simulink model "Joystick"  (R2023a)
settings: Solver=FixedStepDiscrete  StartTime=0.0  StopTime=inf  RelTol=1e-3
values from neighbouring files (symbols this model uses):
  stopSimulationFlag = 0    [InitializeModelForTest.m]
undefined symbols (not defined in the file or in its folder): ComPortTransmitData, NULL, pitchBoundary, rollBoundary, throttleBoundary, yawBoundary
libraries: instrumentseriallib x6, aerolibanimutils x5
settings Model: Creator=admin  LastModifiedBy=ASUS
settings OptimizationCC: DefaultParameterBehavior=Inlined  UseDivisionForNetSlopeComputation=on  GainParamInheritBuiltInType=on  UseFloatMulNetSlope=on  InlineInvariantSignals=on  PassReuseOutputArgsAs=Individual arguments  ZeroExternalMemoryAtStartup=off  ZeroInternalMemoryAtStartup=off  NoFixptDivByZeroProtection=on  EfficientFloat2IntCast=on  LifeSpan=1  OptimizeBlockOrder=speed  DifferentSizesBufferReuse=on  EfficientTunableParamExpr=on
settings DebuggingCC: ParameterTunabilityLossMsg=error  SFUnexpectedBacktrackingDiag=warning  SFNoUnconditionalDefaultTransitionDiag=warning
settings HardwareCC: ProdBitPerPointer=32  ProdBitPerSizeT=32  ProdBitPerPtrDiffT=32  ProdLargestAtomicInteger=Long  ProdLargestAtomicFloat=Double  ProdWordSize=32  ProdLongLongMode=on  ProdHWDeviceType=ARM Compatible->ARM Cortex-M  TargetBitPerPointer=64  TargetBitPerSizeT=64  TargetBitPerPtrDiffT=64  TargetLongLongMode=on  TargetIntDivRoundTo=Zero  TargetEndianess=LittleEndian  TargetWordSize=64  TargetHWDeviceType=MATLAB Host  ProdEqTarget=off
settings SFSimCC: MATLABDynamicMemAlloc=off
settings RTWCC: Description=Embedded Coder  SystemTargetFile=ert.tlc  TemplateMakefile=ert_default_tmf  GenerateReport=on  BuildConfiguration=Debug  LaunchReport=on
settings CodeAppCC: ForceParamTrailComments=on  IgnoreCustomStorageClasses=off  OperatorAnnotations=on  SimulinkDataObjDesc=on  SFDataObjDesc=on  CustomSymbolStrGlobalVar=rt$N$M  CustomSymbolStrType=$N$M  CustomSymbolStrFcn=$N$M$F  CustomSymbolStrMacro=$N$M  InsertBlockDesc=on  EnableCustomComments=on
settings ERTTargetCC: TargetLangStandard=C99 (ISO)  GenerateSampleERTMain=on  IncludeMdlTerminateFcn=off  CombineSignalStateStructs=on  SupportAbsoluteTime=off  SupportComplex=off  SupportNonInlinedSFcns=on  InlinedParameterPlacement=NonHierarchical  ERTCustomFileTemplate=example_file_process.tlc  ERTFilePackagingFormat=CompactWithDataFile

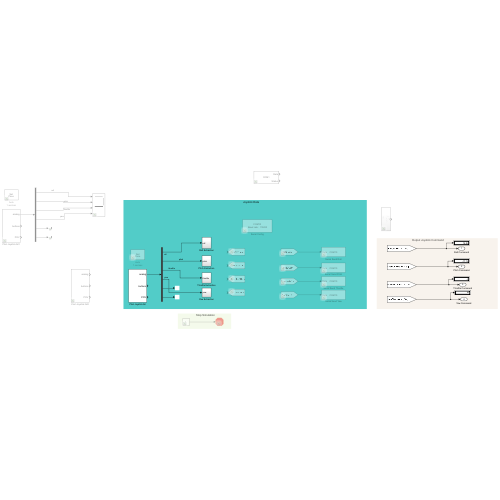
[thumbnail: Simulink's stored preview of the top-level diagram]
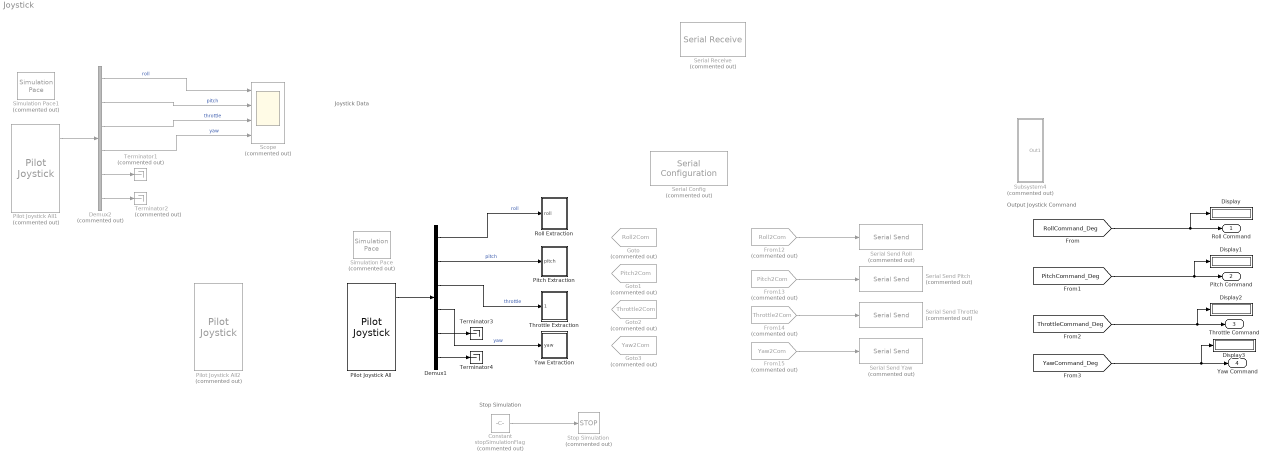
== system Joystick ==
  note: Joystick Data
  note: Output Joystick Command
  note: Stop Simulation
  Constant : Constant  Commented=on  Value=stopSimulationFlag
  Demux1 : Demux  Outputs=6
  Demux2 : Demux  Commented=on  Outputs=6
  Display{,1..3} (4 alike) : Display
  From12 : From  Commented=on  GotoTag=Roll2Com  TagVisibility=global
  From13 : From  Commented=on  GotoTag=Pitch2Com  TagVisibility=global
  From14 : From  Commented=on  GotoTag=Throttle2Com  TagVisibility=global
  From15 : From  Commented=on  GotoTag=Yaw2Com  TagVisibility=global
  Goto : Goto  Commented=on  GotoTag=Roll2Com  TagVisibility=global
  Goto1 : Goto  Commented=on  GotoTag=Pitch2Com  TagVisibility=global
  Goto2 : Goto  Commented=on  GotoTag=Throttle2Com  TagVisibility=global
  Goto3 : Goto  Commented=on  GotoTag=Yaw2Com  TagVisibility=global
  Pilot Joystick All : aerolibanimutils/Pilot Joystick  JoystickID=Joystick1  OutputConfiguration=AllOutputs  SampleTime=1/50
      settings: LibrarySourceBlock=aerolibanimutils/Pilot Joystick All
  Pilot Joystick All1 : aerolibanimutils/Pilot Joystick  Commented=on  JoystickID=Joystick1  OutputConfiguration=AllOutputs  SampleTime=1/50
      settings: LibrarySourceBlock=aerolibanimutils/Pilot Joystick All
  Pilot Joystick All2 : aerolibanimutils/Pilot Joystick  Commented=on  JoystickID=Joystick1  OutputConfiguration=AllOutputs  SampleTime=1/50
      settings: LibrarySourceBlock=aerolibanimutils/Pilot Joystick All
  Pitch Extraction : Subsystem
  Roll Extraction : Subsystem
  Scope : Scope  Commented=on  NumInputPorts=4
  Serial Config : instrumentseriallib/Serial Configuration  Priority=-200000  Commented=on  PortSel=COM10  Port=COM10  ComPort=COM10  BaudRate=115200  DataBits=8  Parity=none  StopBits=1  ByteOrder=little-endian  FlowControl=none  Timeout=10  SimulateUsing=Interpreted execution  BlockInModel=on  aMode=1
  Serial Receive : instrumentseriallib/Serial Receive  Priority=1  Commented=on  PortSel=COM1  Port=COM1  ComPort=COM1  DataType=uint8  SaveDataType=uint8  ToggleHeader=on  Header=[]  ToggleTerminator=on  Terminator=<none>  CustomTerminator=[]  InputFormat=Column major  ToggleDataSize=on  DataSize=[1 1]  EnableBlockingMode=off  ActionDataUnavailable=Output last received value  ActionWhenDataUnavailable=Output last received value  CustomValue=0  SampleTime=0.01  SimulateUsing=Interpreted execution  BlockInModel=on  aMode=1
      settings: LibrarySourceBlock=embeddedtargetslib/Host Communication/Serial Receive
  Serial Send Pitch : instrumentseriallib/Serial Send  Priority=1  Commented=on  PortSel=COM10  Port=COM10  ComPort=COM10  Header=['P']  Terminator=NULL ('\0')  CustomTerminator=[' ']  EnableBlockingMode=off  SimulateUsing=Interpreted execution  BlockInModel=on  aMode=1
  Serial Send Roll : instrumentseriallib/Serial Send  Priority=1  Commented=on  PortSel=COM10  Port=COM10  ComPort=COM10  Header=['R']  Terminator=NULL ('\0')  CustomTerminator=[' ']  EnableBlockingMode=off  SimulateUsing=Interpreted execution  BlockInModel=on  aMode=1
  Serial Send Throttle : instrumentseriallib/Serial Send  Priority=1  Commented=on  PortSel=COM10  Port=COM10  ComPort=COM10  Header=['T']  Terminator=NULL ('\0')  CustomTerminator=[' ']  EnableBlockingMode=off  SimulateUsing=Interpreted execution  BlockInModel=on  aMode=1
  Serial Send Yaw : instrumentseriallib/Serial Send  Priority=1  Commented=on  PortSel=COM10  Port=COM10  ComPort=COM10  Header=['Y']  Terminator=NULL ('\0')  CustomTerminator=[' ']  EnableBlockingMode=off  SimulateUsing=Interpreted execution  BlockInModel=on  aMode=1
  Simulation Pace : aerolibanimutils/Simulation Pace  Commented=on  SimulationPace=1  SleepMode=Auto  OutputPaceError=off  SampleTime=1/50
  Simulation Pace1 : aerolibanimutils/Simulation Pace  Commented=on  SimulationPace=1  SleepMode=Auto  OutputPaceError=off  SampleTime=1/50
  Stop Simulation : Stop  Commented=on
  Subsystem4 : Subsystem  Commented=on
  Terminator1 : Terminator  Commented=on
  Terminator2 : Terminator  Commented=on
  Terminator3 : Terminator
  Terminator4 : Terminator
  Throttle Extraction : Subsystem
  Yaw Extraction : Subsystem
  Roll Command : Outport
  Pitch Command : Outport  Port=2
  Throttle Command : Outport  Port=3
  Yaw Command : Outport  Port=4
  wires:
  Demux1/6 -> Terminator4/1
  Demux1/5 -> Terminator3/1
  Pilot Joystick All/1 -> Demux1/1
  Demux1/2 -> Pitch Extraction/1(pitch)  "pitch"
  Demux1/3 -> Throttle Extraction/1(throttle)  "throttle"
  Demux1/4 -> Yaw Extraction/1(yaw)  "yaw"
  Constant/1 -> Stop Simulation/1
  [PitchCommand_Deg] -> Display1/1, Pitch Command/1
  [ThrottleCommand_Deg] -> Display2/1, Throttle Command/1
  [YawCommand_Deg] -> Display3/1, Yaw Command/1
  [RollCommand_Deg] -> Display/1, Roll Command/1
  From12/1 -> Serial Send Roll/1
  From13/1 -> Serial Send Pitch/1
  From14/1 -> Serial Send Throttle/1
  From15/1 -> Serial Send Yaw/1
  Demux2/4 -> Scope/4  "yaw"
  Demux2/3 -> Scope/3  "throttle"
  Demux2/2 -> Scope/2  "pitch"
  Demux2/1 -> Scope/1  "roll"
  Pilot Joystick All1/1 -> Demux2/1
  Demux2/5 -> Terminator1/1
  Demux2/6 -> Terminator2/1
  Demux1/1 -> Roll Extraction/1(roll)  "roll"

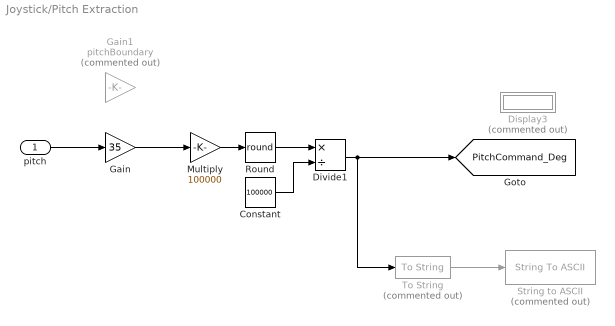
== system Joystick/Pitch Extraction ==
  pitch : Inport
  Constant : Constant  Value=100000
  Display3 : Display  Commented=on
  Divide1 : Product  Inputs=*/
  Gain : Gain  Gain=35
  Gain1 : Gain  Commented=on  Gain=pitchBoundary
  Multiply : Gain  Gain=100000
  Round : Rounding  Operator=round
  String to ASCII : StringToASCII  Commented=on  OutputVectorSize=8
  To String : ToString  Commented=on
  tag scope: PitchCommand_Deg=global
  wires:
  pitch/1 -> Gain/1
  To String/1 -> String to ASCII/1
  Multiply/1 -> Round/1
  Constant/1 -> Divide1/2
  Round/1 -> Divide1/1
  Gain/1 -> Multiply/1
  Divide1/1 -> [PitchCommand_Deg], To String/1

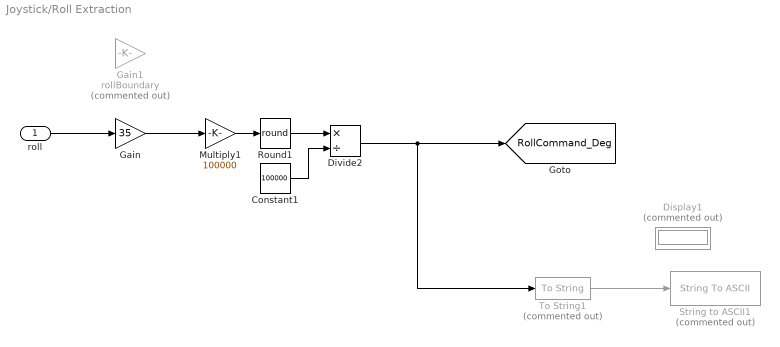
== system Joystick/Roll Extraction ==
  roll : Inport
  Constant1 : Constant  Value=100000
  Display1 : Display  Commented=on
  Divide2 : Product  Inputs=*/
  Gain : Gain  Gain=35
  Gain1 : Gain  Commented=on  Gain=rollBoundary
  Multiply1 : Gain  Gain=100000
  Round1 : Rounding  Operator=round
  String to ASCII1 : StringToASCII  Commented=on  OutputVectorSize=8
  To String1 : ToString  Commented=on
  tag scope: RollCommand_Deg=global
  wires:
  roll/1 -> Gain/1
  Divide2/1 -> [RollCommand_Deg], To String1/1
  Round1/1 -> Divide2/1
  Multiply1/1 -> Round1/1
  Constant1/1 -> Divide2/2
  To String1/1 -> String to ASCII1/1
  Gain/1 -> Multiply1/1

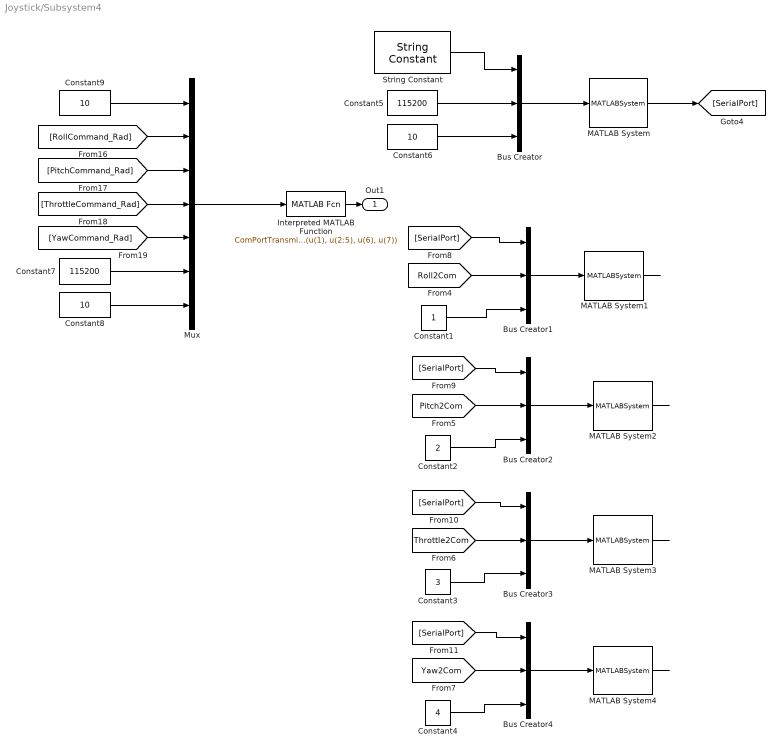
== system Joystick/Subsystem4 ==
  Bus Creator{,1..4} (5 alike) : BusCreator  Inputs=3
  Constant1 : Constant
  Constant2 : Constant  Value=2
  Constant3 : Constant  Value=3
  Constant4 : Constant  Value=4
  Constant5 : Constant  Value=115200
  Constant6 : Constant  Value=10
  Constant7 : Constant  Value=115200
  Constant8 : Constant  Value=10
  Constant9 : Constant  Value=10
  Interpreted MATLAB Function : MATLABFcn  MATLABFcn=ComPortTransmitData(u(1), u(2:5), u(6), u(7))
  MATLAB System : MATLABSystem  System=PortConfig  SimulateUsing=Code generation
      mask Type: PortConfig
      mask Display:
      | disp('PortConfig');
      | port_label('input',1,'u');
      | port_label('output',1,'y');
  MATLAB System{1..4} (4 alike) : MATLABSystem  System=SerialSend  SimulateUsing=Code generation
      mask Type: SerialSend
      mask Display:
      | disp('SerialSend');
      | port_label('input',1,'u');
      | port_label('output',1,'y');
  Mux : Mux  Inputs=7
  String Constant : StringConstant  String="\"COM10\""
  Out1 : Outport
  wires:
  [Yaw2Com] -> Bus Creator4/2
  Constant5/1 -> Bus Creator/2
  [PitchCommand_Rad] -> Mux/3
  MATLAB System4/1 -> ?
  [SerialPort] -> Bus Creator3/1
  Interpreted MATLAB Function/1 -> Out1/1
  Bus Creator2/1 -> MATLAB System2/1
  [Roll2Com] -> Bus Creator1/2
  Constant4/1 -> Bus Creator4/3
  Bus Creator/1 -> MATLAB System/1
  [SerialPort] -> Bus Creator4/1
  Bus Creator1/1 -> MATLAB System1/1
  [SerialPort] -> Bus Creator2/1
  MATLAB System1/1 -> ?
  MATLAB System3/1 -> ?
  [Throttle2Com] -> Bus Creator3/2
  Constant8/1 -> Mux/7
  MATLAB System/1 -> [SerialPort]
  String Constant/1 -> Bus Creator/1
  [RollCommand_Rad] -> Mux/2
  Bus Creator4/1 -> MATLAB System4/1
  Mux/1 -> Interpreted MATLAB Function/1
  Constant9/1 -> Mux/1
  Constant6/1 -> Bus Creator/3
  Bus Creator3/1 -> MATLAB System3/1
  MATLAB System2/1 -> ?
  Constant2/1 -> Bus Creator2/3
  Constant1/1 -> Bus Creator1/3
  Constant7/1 -> Mux/6
  [Pitch2Com] -> Bus Creator2/2
  [YawCommand_Rad] -> Mux/5
  [ThrottleCommand_Rad] -> Mux/4
  Constant3/1 -> Bus Creator3/3
  [SerialPort] -> Bus Creator1/1

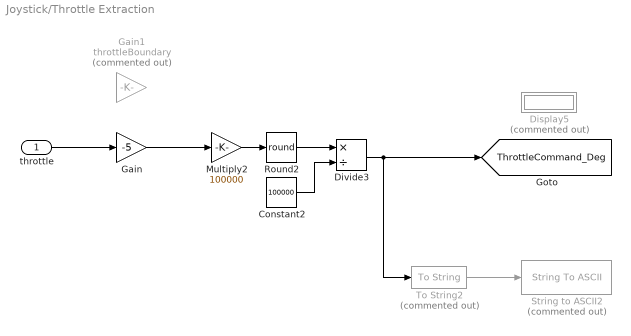
== system Joystick/Throttle Extraction ==
  throttle : Inport
  Constant2 : Constant  Value=100000
  Display5 : Display  Commented=on
  Divide3 : Product  Inputs=*/
  Gain : Gain  Gain=-5
  Gain1 : Gain  Commented=on  Gain=throttleBoundary
  Multiply2 : Gain  Gain=100000
  Round2 : Rounding  Operator=round
  String to ASCII2 : StringToASCII  Commented=on  OutputVectorSize=8
  To String2 : ToString  Commented=on
  tag scope: ThrottleCommand_Deg=global
  wires:
  Multiply2/1 -> Round2/1
  To String2/1 -> String to ASCII2/1
  Divide3/1 -> [ThrottleCommand_Deg], To String2/1
  Constant2/1 -> Divide3/2
  Round2/1 -> Divide3/1
  throttle/1 -> Gain/1
  Gain/1 -> Multiply2/1

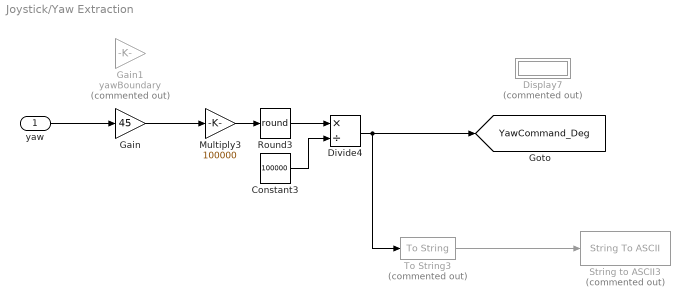
== system Joystick/Yaw Extraction ==
  yaw : Inport
  Constant3 : Constant  Value=100000
  Display7 : Display  Commented=on
  Divide4 : Product  Inputs=*/
  Gain : Gain  Gain=45
  Gain1 : Gain  Commented=on  Gain=yawBoundary
  Multiply3 : Gain  Gain=100000
  Round3 : Rounding  Operator=round
  String to ASCII3 : StringToASCII  Commented=on  OutputVectorSize=8
  To String3 : ToString  Commented=on
  tag scope: YawCommand_Deg=global
  wires:
  Multiply3/1 -> Round3/1
  Divide4/1 -> [YawCommand_Deg], To String3/1
  Constant3/1 -> Divide4/2
  To String3/1 -> String to ASCII3/1
  Round3/1 -> Divide4/1
  yaw/1 -> Gain/1
  Gain/1 -> Multiply3/1
